simulink model "BatchComputeVariance"  (R2016b)
settings: Solver=FixedStepDiscrete  StartTime=0.0  StopTime=inf  FixedStep=sCoreParams.core.stepPeriod  RelTol=1e-3
undefined symbols (not defined in the file): sCoreParams, sCoreParams_decoders_txDetector_overrideTXbool, sCoreParams_decoders_txDetector_overrideTXval, sCoreParams_decoders_txDetector_realTimeUpdateThreshold
libraries: simulink x3
settings Model: DataTypeOverride=Double  MinMaxOverflowLogging=ForceOff  Creator=anish  LastModifiedBy=rzelmann
settings SolverCC: EnableConcurrentExecution=on
settings DataIOCC: LimitDataPoints=on  SaveFormat=Array  SignalLoggingSaveFormat=ModelDataLogs
settings OptimizationCC: BlockReduction=off  BooleanDataType=off  DefaultParameterBehavior=Inlined  OptimizeBlockIOStorage=off  BufferReuse=off  GlobalBufferReuse=off  ExpressionFolding=off  LocalBlockOutputs=off  LifeSpan=inf
settings DebuggingCC: SaveWithParameterizedLinksMsg=none  SignalResolutionControl=TryResolveAllWithWarning  MultiTaskDSMMsg=warning  MultiTaskCondExecSysMsg=none  StateNameClashWarn=warning  SFUnexpectedBacktrackingDiag=warning  SFNoUnconditionalDefaultTransitionDiag=warning  SFExecutionAtInitializationDiag=none
settings HardwareCC: ProdBitPerPointer=32  ProdBitPerSizeT=32  ProdBitPerPtrDiffT=32  ProdLargestAtomicFloat=None  ProdWordSize=32  ProdLongLongMode=on  ProdHWDeviceType=Generic->32-bit x86 compatible  TargetBitPerPointer=64  TargetBitPerSizeT=64  TargetBitPerPtrDiffT=64  TargetLongLongMode=on  TargetIntDivRoundTo=Zero  TargetEndianess=LittleEndian  TargetWordSize=64  TargetHWDeviceType=MATLAB Host
settings RTWCC: SystemTargetFile=slrt.tlc  TemplateMakefile=slrt_default_tmf  Description=Simulink Real-Time  RTWCompilerOptimization=on
settings ConfigComp: CovMetricSettings=dw  CovHtmlReporting=on  CovSaveCumulativeToWorkspaceVar=on  CovSaveSingleToWorkspaceVar=on  CovExternalEMLEnable=off

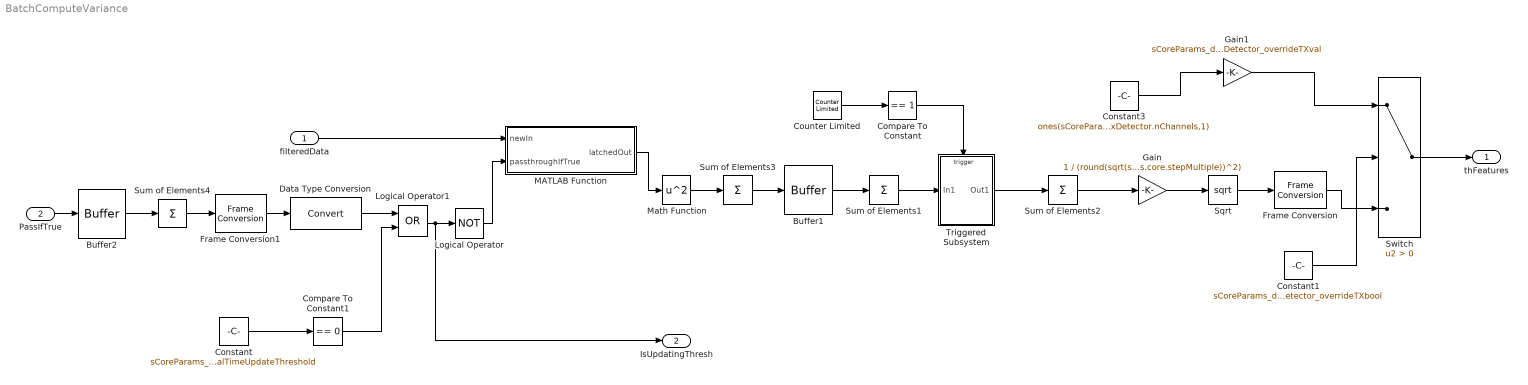
== system BatchComputeVariance ==
  filteredData : Inport  PortDimensions=[sCoreParams.FrameSize sCoreParams.decoders.txDetector.nChannels]  SampleTime=sCoreParams.core.stepPeriod  Interpolate=off
  PassIfTrue : Inport  Port=2  OutDataTypeStr=boolean
  Buffer1 : Buffer  N=round(sqrt(sCoreParams.core.stepMultiple))  V=round(sqrt(sCoreParams.core.stepMultiple)) - 1  TreatMby1Signals=One channel
  Buffer2 : Buffer  N=200  V=199  TreatMby1Signals=One channel
  Compare To Constant : simulink/Logic and Bit Operations/Compare To Constant  relop===  const=1  OutDataTypeStr=boolean
  Compare To Constant1 : simulink/Logic and Bit Operations/Compare To Constant  relop===  const=0  OutDataTypeStr=boolean
  Constant : Constant  Value=sCoreParams_decoders_txDetector_realTimeUpdateThreshold
  Constant1 : Constant  Value=sCoreParams_decoders_txDetector_overrideTXbool
  Constant3 : Constant  Value=ones(sCoreParams.decoders.txDetector.nChannels,1)
  Counter Limited : simulink/Sources/Counter Limited  uplimit=round(sqrt(sCoreParams.core.stepMultiple))  tsamp=-1
  Data Type Conversion : DataTypeConversion
  Frame Conversion : FrameConversion  InheritSamplingMode=off  OutFrame=Sample-based
  Frame Conversion1 : FrameConversion  InheritSamplingMode=off  OutFrame=Sample-based
  Gain : Gain  Gain=1 / (round(sqrt(sCoreParams.core.stepMultiple))^2)
  Gain1 : Gain  Gain=sCoreParams_decoders_txDetector_overrideTXval
  Logical Operator : Logic  Operator=NOT  AllPortsSameDT=off  OutDataTypeStr=boolean
  Logical Operator1 : Logic  Operator=OR  AllPortsSameDT=off  OutDataTypeStr=boolean
  MATLAB Function : MATLAB Function  TreatAsAtomicUnit=on
  Math Function : Math  Operator=square  SaturateOnIntegerOverflow=on
  Sqrt : Sqrt  SaturateOnIntegerOverflow=on
  Sum of Elements1 : Sum  Inputs=+  CollapseMode=Specified dimension
  Sum of Elements2 : Sum  Inputs=+  CollapseMode=Specified dimension
  Sum of Elements3 : Sum  Inputs=+  CollapseMode=Specified dimension
  Sum of Elements4 : Sum  Inputs=+
  Switch : Switch  Criteria=u2 > Threshold
  Triggered Subsystem : Subsystem  TreatAsAtomicUnit=on
  thFeatures : Outport
  IsUpdatingThresh : Outport  Port=2
  wires:
  Math Function/1 -> Sum of Elements3/1
  Buffer1/1 -> Sum of Elements1/1
  Sum of Elements3/1 -> Buffer1/1
  Sum of Elements1/1 -> Triggered Subsystem/1(In1)
  Gain/1 -> Sqrt/1
  Sqrt/1 -> Frame Conversion/1
  Sum of Elements2/1 -> Gain/1
  Counter Limited/1 -> Compare To Constant/1
  Compare To Constant/1 -> Triggered Subsystem/Trigger
  Triggered Subsystem/1(Out1) -> Sum of Elements2/1
  PassIfTrue/1 -> Buffer2/1
  Logical Operator/1 -> MATLAB Function/2(passthroughIfTrue)
  filteredData/1 -> MATLAB Function/1(newIn)
  MATLAB Function/1(latchedOut) -> Math Function/1
  Buffer2/1 -> Sum of Elements4/1
  Sum of Elements4/1 -> Frame Conversion1/1
  Frame Conversion1/1 -> Data Type Conversion/1
  Logical Operator1/1 -> Logical Operator/1, IsUpdatingThresh/1
  Data Type Conversion/1 -> Logical Operator1/1
  Constant/1 -> Compare To Constant1/1
  Compare To Constant1/1 -> Logical Operator1/2
  Constant3/1 -> Gain1/1
  Constant1/1 -> Switch/2
  Frame Conversion/1 -> Switch/3
  Gain1/1 -> Switch/1
  Switch/1 -> thFeatures/1

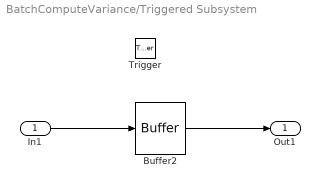
== system BatchComputeVariance/Triggered Subsystem ==
  In1 : Inport
  Trigger : TriggerPort  VariantControl=Variant
  Buffer2 : Buffer  N=round(sqrt(sCoreParams.core.stepMultiple))  V=round(sqrt(sCoreParams.core.stepMultiple)) - 1  TreatMby1Signals=One channel
  Out1 : Outport
  wires:
  In1/1 -> Buffer2/1
  Buffer2/1 -> Out1/1

== matlab function BatchComputeVariance/MATLAB Function ==
  data: newIn input; latchedOut output; passthroughIfTrue input
function latchedOut = FlipFlop(newIn,passthroughIfTrue)
%#codegen

persistent latchedSignal

if isempty(latchedSignal)
    latchedSignal = newIn;
end

if passthroughIfTrue
    latchedSignal = newIn;
end

latchedOut = latchedSignal;

end
